simulink model "BALLBOT_1"  (R2015a)
settings: Solver=ode45  SolverMode=SingleTasking  StartTime=0  StopTime=50  MaxStep=0.001  RelTol=1e-3  AbsTol=1e-6
InitFcn:
  | parametros;
StartFcn:
  | %vrview('Ballbot2')
StopFcn:
  | % Se selecionar velocidade, tirar o comentário abaixo
  | %gerarPlotVel;
  | % Se selecionar posição, tirar o comentário abaixo
  | gerarPlotPos;
values from neighbouring files (symbols this model uses):
  g = 9.81    [parametros.m]
  Ic = 0.024    [parametros.m]
  L = 0.2    [parametros.m]
  Mc = 1.6    [parametros.m]
  Mr = 0.5    [parametros.m]
  r = 0.12    [parametros.m]
undefined symbols (not defined in the file or in its folder): K
settings Model: ExtModeAutoUpdateStatusClock=off  Creator=The MathWorks Inc.  LastModifiedBy=Pedro
settings DataIOCC: ExternalInput=[]  InitialState=[]  LimitDataPoints=off  SignalLoggingSaveFormat=ModelDataLogs  SaveOutput=off  SaveTime=off
settings OptimizationCC: BlockReduction=off  BooleanDataType=off  BufferReuse=off  ExpressionDepthLimit=2147483647  InitFltsAndDblsToZero=on
settings DebuggingCC: AlgebraicLoopMsg=none  SaveWithParameterizedLinksMsg=none  UnderspecifiedInitializationDetection=Classic  MergeDetectMultiDrivingBlocksExec=none  SignalResolutionControl=TryResolveAllWithWarning  MultiTaskDSMMsg=warning  MultiTaskCondExecSysMsg=none  SigSpecEnsureSampleTimeMsg=none  FcnCallInpInsideContextMsg=UseLocalSettings  UnconnectedInputMsg=none  UnconnectedOutputMsg=none  UnconnectedLineMsg=none  StateNameClashWarn=warning
settings HardwareCC: TargetLongLongMode=on  TargetIntDivRoundTo=Zero  TargetEndianess=LittleEndian  TargetHWDeviceType=MATLAB Host  ProdEqTarget=off
settings GRTTargetCC: TargetFcnLib=ansi_tfl_tmw.mat  CombineOutputUpdateFcns=off  GRTInterface=on

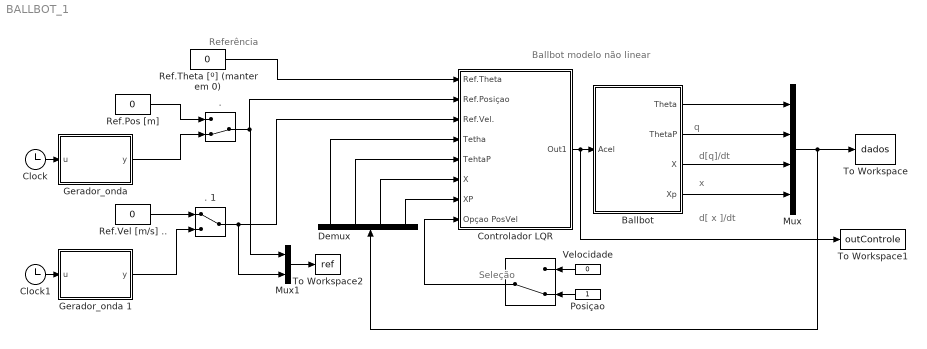
== system BALLBOT_1 ==
  note: Ballbot modelo não linear
  note: Referência
  note: Seleção
  note: x
  note: d[ x ]/dt
  note: q
  note: d[q]/dt
  " " : ManualSwitch  CurrentSetting=0
  " . " : ManualSwitch  CurrentSetting=0
  " . 1" : ManualSwitch
  Ballbot : Subsystem  mask(Ballbot){thetac0=0}
      mask prompts: thetac0 "Ângulo inicial do corpo (graus)"
      mask help:
      | Modelo dinâmico não-linear do Ballbot.
      | Selecione "Look Under Mask" para ver o diagrama de simulação.
      mask Help: Unmask and double-click to see dynamics.
      mask Display: image(imread('ballbot_LMI.png'));
  Clock : Clock
  Clock1 : Clock
  Controlador LQR : Subsystem
      mask Display:
      | image(imread('ArduinoMega.png'));
      | 
      | 
      | 
      | port_label('output', 1, 'Acel Ang.');
      | 
      | port_label('input', 1, 'Ref.Theta');
      | port_label('input', 2, 'Ref.Pos.');
      | port_label('input', 3, 'Ref.Vel.');
      | port_label('input', 4, 'Theta');
      | port_label('input', 5, 'ThetaP');
      | port_label('input', 6, 'X');
      | port_label('input', 7, 'XP');
      | 
      | port_label('input', 8, 'Opção Pos.Vel');
  Demux : Demux
  "Gerador_onda " : MATLAB Function  TreatAsAtomicUnit=on
  Gerador_onda 1 : MATLAB Function  TreatAsAtomicUnit=on
  Mux : Mux
  Mux1 : Mux  Inputs=2
  Posiçao : Constant
  "Ref.Pos [m] " : Constant  Value=0
  Ref.Theta [º] (manter em 0) : Constant  Value=0
  Ref.Vel [m/s] .. : Constant  Value=0
  To Workspace : ToWorkspace  VariableName=dados  SaveFormat=Structure With Time  SampleTime=-1
  To Workspace1 : ToWorkspace  VariableName=outControle  SaveFormat=Structure With Time  SampleTime=-1
  To Workspace2 : ToWorkspace  VariableName=ref  SaveFormat=Structure With Time  SampleTime=-1
  Velocidade : Constant  Value=0
  wires:
  Ballbot/1(Theta) -> Mux/1
  Ballbot/2(ThetaP) -> Mux/2
  Ballbot/4(Xp) -> Mux/4
  Ref.Theta [º] (manter em 0)/1 -> Controlador LQR/1(Ref.Theta)
  Demux/1 -> Controlador LQR/4(Tetha)
  Demux/2 -> Controlador LQR/5(TehtaP)
  Demux/3 -> Controlador LQR/6(X)
  Demux/4 -> Controlador LQR/7(XP)
  Mux/1 -> Demux/1, To Workspace/1
  Velocidade/1 -> " "/1
  Posiçao/1 -> " "/2
  " "/1 -> Controlador LQR/8(Opçao PosVel)
  Controlador LQR/1(Out1) -> To Workspace1/1, Ballbot/1(Acel)
  Ballbot/3(X) -> Mux/3
  Mux1/1 -> To Workspace2/1
  " . "/1 -> Controlador LQR/2(Ref.Posiçao), Mux1/1
  "Ref.Pos [m] "/1 -> " . "/1
  Clock/1 -> "Gerador_onda "/1(u)
  Clock1/1 -> Gerador_onda 1/1(u)
  Ref.Vel [m/s] ../1 -> " . 1"/1
  Gerador_onda 1/1(y) -> " . 1"/2
  " . 1"/1 -> Controlador LQR/3(Ref.Vel.), Mux1/2
  "Gerador_onda "/1(y) -> " . "/2

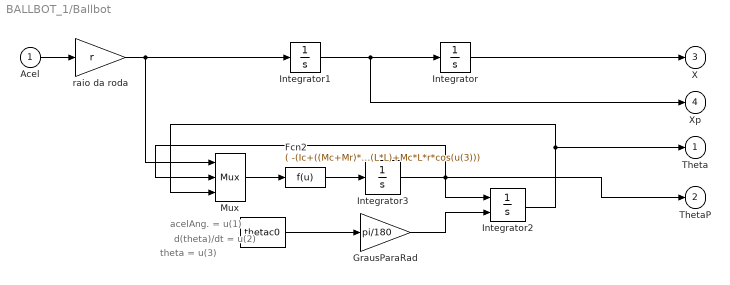
== system BALLBOT_1/Ballbot ==
  note: theta = u(3)
  note: d(theta)/dt = u(2)
  note: acelAng. = u(1)
  Acel : Inport
  "   " : Constant  Value=thetac0
  Fcn2 : Fcn  Expr=( -(Ic+((Mc+Mr)*r*r)+Mc*L*r*cos(u(3)))*u(1) + Mc*g*L*sin(u(3))+Mc*r*L*u(2)*u(2)*sin(u(3)))/ (Ic+Mc*(L*L)+Mc*L*r*cos(u(3)))
  "GrausParaRad " : Gain  Gain=pi/180
  Integrator : Integrator
  Integrator1 : Integrator
  Integrator2 : Integrator  InitialConditionSource=external
  Integrator3 : Integrator
  Mux : Mux  Inputs=3
  raio da roda : Gain  Gain=r
  Theta : Outport
  ThetaP : Outport  Port=2
  X : Outport  Port=3
  Xp : Outport  Port=4
  wires:
  Fcn2/1 -> Integrator3/1
  Mux/1 -> Fcn2/1
  Integrator2/1 -> Mux/3, Theta/1
  "   "/1 -> "GrausParaRad "/1
  "GrausParaRad "/1 -> Integrator2/2
  Integrator3/1 -> Mux/2, ThetaP/1, Integrator2/1
  Integrator/1 -> X/1
  Integrator1/1 -> Xp/1, Integrator/1
  Acel/1 -> raio da roda/1
  raio da roda/1 -> Integrator1/1, Mux/1

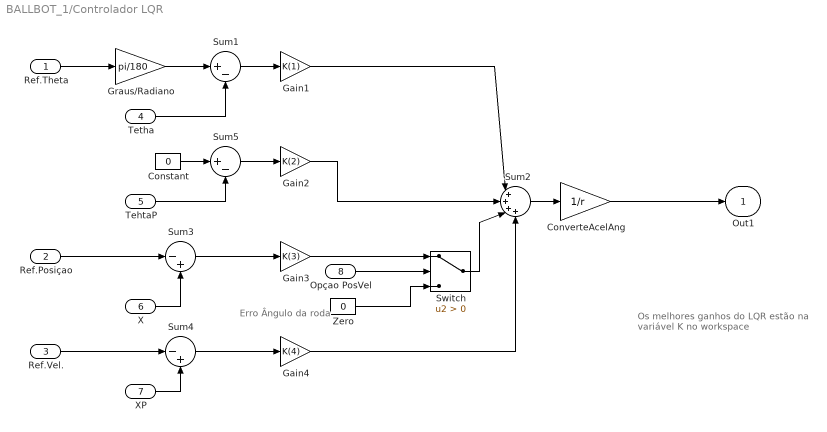
== system BALLBOT_1/Controlador LQR ==
  note: Os melhores ganhos do LQR estão na variável K no workspace
  note: Erro
      | Ângulo da roda
  Ref.Theta : Inport
  Ref.Posiçao : Inport  Port=2
  Ref.Vel. : Inport  Port=3
  Tetha : Inport  Port=4
  TehtaP : Inport  Port=5
  X : Inport  Port=6
  XP : Inport  Port=7
  Opçao PosVel : Inport  Port=8
  Constant : Constant  Value=0
  ConverteAcelAng : Gain  Gain=1/r
  Gain1 : Gain  Gain=K(1)
  Gain2 : Gain  Gain=K(2)
  Gain3 : Gain  Gain=K(3)
  Gain4 : Gain  Gain=K(4)
  Graus/Radiano : Gain  Gain=pi/180
  Sum1 : Sum  Inputs=|+-
  Sum2 : Sum  Inputs=|++++
  Sum3 : Sum  Inputs=|-+
  Sum4 : Sum  Inputs=|-+
  Sum5 : Sum  Inputs=|+-
  Switch : Switch  Criteria=u2 > Threshold
  Zero : Constant  Value=0
  Out1 : Outport
  wires:
  Gain1/1 -> Sum2/1
  Gain2/1 -> Sum2/2
  Gain4/1 -> Sum2/4
  Ref.Theta/1 -> Graus/Radiano/1
  Tetha/1 -> Sum1/2
  Sum1/1 -> Gain1/1
  Graus/Radiano/1 -> Sum1/1
  Opçao PosVel/1 -> Switch/2
  Gain3/1 -> Switch/1
  Switch/1 -> Sum2/3
  Zero/1 -> Switch/3
  Sum5/1 -> Gain2/1
  TehtaP/1 -> Sum5/2
  Constant/1 -> Sum5/1
  Ref.Posiçao/1 -> Sum3/1
  X/1 -> Sum3/2
  Ref.Vel./1 -> Sum4/1
  XP/1 -> Sum4/2
  Sum3/1 -> Gain3/1
  Sum4/1 -> Gain4/1
  Sum2/1 -> ConverteAcelAng/1
  ConverteAcelAng/1 -> Out1/1

== matlab function BALLBOT_1/Gerador_onda 1 ==
  data: y output; u input
function y = fcn(u)
%#codegen
y=0;

if u>0
    y=0.1;
end
if u>20
    y=0;
end
if u>40
    y=-0.1;
end
if u>60
    y=0;
end

== matlab function BALLBOT_1/Gerador_onda  ==
  data: y output; u input
function y = fcn(u)
%#codegen
%{
y=0;

if u>0
    y=0.4;
end
if u>20
    y=0;
end
if u>40
    y=-0.4;
end
if u>60
    y=0;
%}  
    

  y=u*0.1;
  if y>2
    y=2;
  end
  
  
  
    
end
